simulink library "DiSC_ToolboxOpal_V12"  (R2012b)
settings: Solver=ode45  StartTime=0.0  StopTime=10.0  RelTol=1e-3
undefined symbols (not defined in the file or in its folder): SamplingTime
(part 1 of 5)
settings Model: Creator=mos  LastModifiedBy=smartgrid

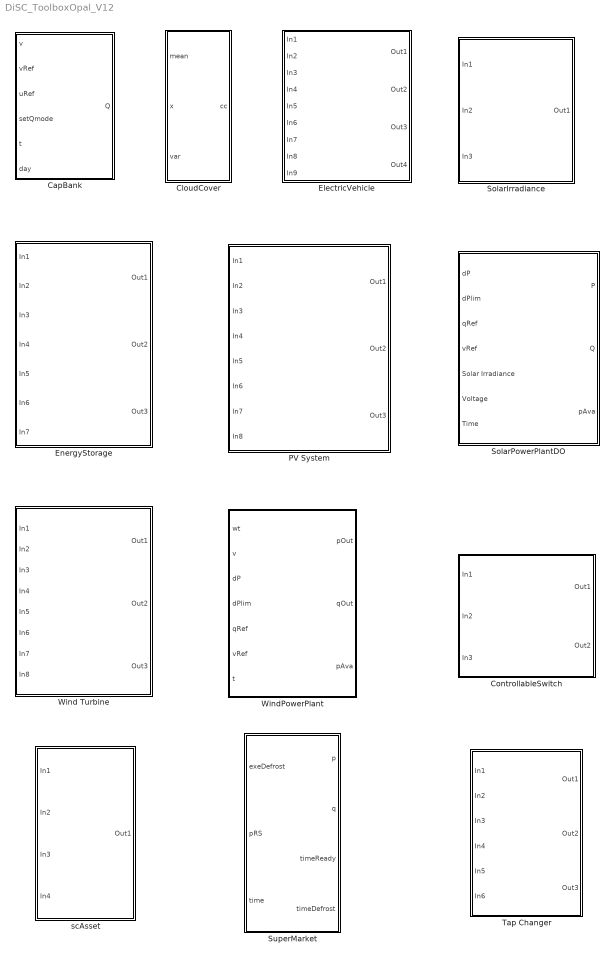
== system DiSC_ToolboxOpal_V12 ==
  CapBank : Subsystem  TreatAsAtomicUnit=on  SystemSampleTime=60
      mask help:
      | % A simulink version of cbAsset module using embedded matlab function
      |     % block on Simulink
      |     %   The cbAsset can be controlled to inject reactive power into the
      |     %   grid in steps. It is characterized by having a number of steps and
      |     %   a reactive output per step (i.e., it can inject from 0 - Qmax in
      |     %   N steps).
      |     %
      |     %
      |     % Revision:
      |     % 15-10-2014, R. Pedersen, Aalborg University. Notes:
      |     % 29-11-2014, R. Olsen/M. Kemal, Aalborg University (Simulink)
      |     % 20-06-2015, F. Iov/M. Kemal, Aalborg University (Simulink toolbox for OPAL)
      |
      |         % Input:
      |             %   - v [V], is the voltage at the connection point.
      |             %   - qRef [VAR], is the reference to active power.
      |             %   - vRef [V], is the voltage reference for the droop control.
      |             %   - uRef [V], is the tap reference
      |             %   - SetQmode will set the reactive power control  mode
      |             %
      |             % Output:
      |             %   - q [VAR], is the reactive power output
      mask Help:
      | % A simulink version of cbAsset module using embedded matlab function
      |     % block on Simulink
      |     %   The cbAsset can be controlled to inject reactive power into the
      |     %   grid in steps. It is characterized by having a number of steps and
      |     %   a reactive output per step (i.e., it can inject from 0 - Qmax in
      |     %   N steps).
      |     %
      |     %
      |     % Revision:
      |     % 15-10-2014, R. Pedersen, Aalborg University. Notes:
      |     % 29-11-2014, R. Olsen/M. Kemal, Aalborg University (Simulink)
      | 
      |         % Input:
      |             %   - v [V], is the voltage at the connection point.
      |             %   - qRef [VAR], is the reference to active power.
      |             %   - vRef [V], is the voltage reference for the droop control.
      |             %
      |             % Output:
      |             %   - q [VAR], is the reactive power output
      mask Display:
      | %%image(imread('cbAsset1.jpg'))
      | port_label('output',1,'q')
      | port_label('input',1,'qRef')
      | port_label('input',2,'vRef')
      | port_label('input',3,'uRef')
      | port_label('input',4,'SetQmode')
      | port_label('input',5,'t')
      | port_label('input',6,'day')
  CloudCover : Subsystem  TreatAsAtomicUnit=on  SystemSampleTime=60
      mask help:
      | %MATLAB embedded block  for OPAL-RT
      |     %
      |     %   The cloud cover model can be used to investigate the behavior
      |     %   of e.g., photovoltaic systems. This model can be used together with
      |     %   the solar irradiance model.
      |     %
      |     %   The model is based on the work by
      |     %   Heinriich Morf (1998-2013)
      |     %
      |     % Revision:
      |     % R. Pedersen, Aalborg University.
      |     % 29-11-2014, R. Olsen/M. Kemal, Aalborg University (Simulink)
      |     % 20-06-2015, F. Iov/M. Kemal, Aalborg University (Simulink toolbox for OPAL)
      mask Help:
      | %MATLAB embedded block  for OPAL-RT
      |     %
      |     %   The cloud cover model can be used to investigate the behavior
      |     %   of e.g., photovoltaic systems. This model can be used together with
      |     %   the solar irradiance model.
      |     %
      |     %   The model is based on the work by
      |     %   Heinriich Morf (1998-2013)
      |     %
      |     % Revision:
      |     % R. Pedersen, Aalborg University.
      |     % 29-11-2014, R. Olsen/M. Kemal, Aalborg University (Simulink)
      |     % 20-06-2015, F. Iov/M. Kemal, Aalborg University (Simulink toolbox for OPAL)
      mask Display:
      | %image(imread('cloudCover.jpg'))
      | port_label('output',1,'cc')
      | port_label('input',1,'mean')
      | port_label('input',2,'var')
      | port_label('input',3,'x')
  ControllableSwitch : Subsystem  TreatAsAtomicUnit=on  SystemSampleTime=60
      mask help:
      | %#codegen
      |     % A Simulink implementation of swAsset using embedded MATLAB function
      |     %%swAsset implements a controllable switch.
      |     %   The swAsset can change the switch position between open and closed.
      |     %   The switch is used to change the electrical grid topology.
      |     %   To ensure realistic simulation scenarios a minimum time between
      |     %   switch state change has been incorporated, along with a maximum
      |     %   number of state changes per day.
      |     %
      |     %   The model is intended for studying voltage control problems and
      |     %   power loss minimization. The switch works by inserting an
      |     %   admittance into the admittance matrix whenever the switch state is
      |     %   closed.
      |     %
      |     % R. Pedersen 05-9-2014, Aalborg University
      |     % 20-06-2015, F. Iov/M. Kemal, Aalborg University (Simulink toolbox for OPAL)
      |     % This template includes the minimum set of functions required
      |     % to define a System object with discrete state.
      |
      |
      |             % Input:
      |             %   - uRef [-], is the reference to switch state (0=open, 1=closed).
      |             %   - k [-], is the sample.
      |             %   - day [-], is the day of the simulation (1-365).
      |             %
      |             % Output:
      |             %   - state [-], is the state of the switch, either open or closed.
      |             %   - y [-], is the admittance to be put into the grid admittance matrix.
      |
      |             % If day changes reset the number of switches a day
      mask Help:
      | %#codegen
      |     % A Simulink implementation of swAsset using embedded MATLAB function
      |     %%swAsset implements a controllable switch.
      |     %   The swAsset can change the switch position between open and closed.
      |     %   The switch is used to change the electrical grid topology.
      |     %   To ensure realistic simulation scenarios a minimum time between
      |     %   switch state change has been incorporated, along with a maximum
      |     %   number of state changes per day.
      |     %
      |     %   The model is intended for studying voltage control problems and
      |     %   power loss minimization. The switch works by inserting an
      |     %   admittance into the admittance matrix whenever the switch state is
      |     %   closed.
      |     %
      |     % R. Pedersen 05-9-2014, Aalborg University
      |     % 20-06-2015, F. Iov/M. Kemal, Aalborg University (Simulink toolbox for OPAL)
      |     % This template includes the minimum set of functions required
      |     % to define a System object with discrete state.
      | 
      | 
      |             % Input:
      |             %   - uRef [-], is the reference to switch state (0=open, 1=closed).
      |             %   - k [-], is the sample.
      |             %   - day [-], is the day of the simulation (1-365).
      |             %
      |             % Output:
      |             %   - state [-], is the state of the switch, either open or closed.
      |             %   - y [-], is the admittance to be put into the grid admittance matrix.
      | 
      |             % If day changes reset the number of switches a day
      mask Display:
      | %image(imread('images\switch.jpg'))
      | port_label('output',1,'state')
      | port_label('output',2,'y')
      | port_label('input',1,'uRef')
      | port_label('input',2,'day')
      | port_label('input',3,'t')
  ElectricVehicle : Subsystem  TreatAsAtomicUnit=on  SystemSampleTime=60
      mask help:
      | % evAsset implements a simple electrical vehicel mobility- and battery model in Simulink.
      |     %   The active power consumption of the battery charging cycle can be
      |     %   controlled when ever the electrical vehical is available at
      |     %   a household charging spot.
      |     %   To simulate when the electrical vehical is available data from the
      |     %   National Travel Survey from Great Britain is used.
      |     %
      |     %   To model the battery a simple first order model of an energy
      |     %   storages is used. The batterys state of charges, when arriving at a
      |     %   charging station/spot, is dependent on the trip the car has conducted.
      |     %
      |     %
      |     % Revision:
      |     % 16-07-2014, C.E. Sloth and R. Pedersen, Aalborg University. Notes:
      |     % 29-11-2014, R. Olsen/M. Kemal, Aalborg University (Simulink)
      |     % 20-06-2015, F. Iov/M. Kemal, Aalborg University (Simulink toolbox for OPAL)
      |             % Input:
      |             %   - k [-], is the sample number.
      |             %   - day [day number], is the day of the year 1-365.
      |             %   - v [-], is the voltage at the connection point.
      |             %   - pRef [W], is the reference to active power.
      |             %   - qRef [VAR], is the reference to reactive power.
      |             %   - vRef [V], is the voltage reference.
      |             %
      |             % Output:
      |             %   - p [W], is the active power output.
      |             %   - q [VAR], is the reactive power output.
      |             %   - e [J], is the EV batery energy level.
      |             %   - away [-]. Indicates if the EV is available for charging.
      |
      |             % If day changes calculate when EV is away from home and how
      |             % much the state of charge has changed.
      mask Help:
      | % evAsset implements a simple electrical vehical mobility- and battery model in Simulink.
      |     %   The active power consumption of the battery charging cycle can be
      |     %   controlled when ever the electrical vehical is available at
      |     %   a household charging spot.
      |     %   To simulate when the electrical vehical is available data from the
      |     %   National Travel Survey from Great Britain is used.
      |     %
      |     %   To model the battery a simple first order model of an energy
      |     %   storages is used. The batterys state of charges, when arriving at a
      |     %   charging station/spot, is dependent on the trip the car has conducted.
      |     %
      |     %
      |     % Revision:
      |     % 16-07-2014, C.E. Sloth and R. Pedersen, Aalborg University. Notes:
      |     % 29-11-2014, R. Olsen/M. Kemal, Aalborg University (Simulink)
      |     % 20-06-2015, F. Iov/M. Kemal, Aalborg University (Simulink toolbox for OPAL)
      |             % Input:
      |             %   - k [-], is the sample number.
      |             %   - day [day number], is the day of the year 1-365.
      |             %   - v [-], is the voltage at the connection point.
      |             %   - pRef [W], is the reference to active power.
      |             %   - qRef [VAR], is the reference to reactive power.
      |             %   - vRef [V], is the voltage reference.
      |             %
      |             % Output:
      |             %   - p [W], is the active power output.
      |             %   - q [VAR], is the reactive power output.
      |             %   - e [J], is the EV batery energy level.
      |             %   - away [-]. Indicates if the EV is available for charging.
      | 
      |             % If day changes calculate when EV is away from home and how
      |             % much the state of charge has changed.
      mask Display:
      | %image(imread( 'electricVehicle.jpg'))
      | port_label( 'output',1, 'p')
      | port_label( 'output',2, 'q')
      | port_label( 'output',3, 'e')
      | port_label( 'output',4, 'away')
      | 
      | port_label( 'input',1, 'day')
      | port_label( 'input',2, 'vMeas')
      | port_label( 'input',3, 'pRef')
      | port_label( 'input',4, 'pMode')
      | port_label( 'input',5, 'qRef')
      | port_label( 'input',6, 'qMode')
      | port_label( 'input',7, 'vRef')
      | port_label( 'input',8, 'time')
      | port_label( 'input',9, 'seed')
  EnergyStorage : Subsystem  TreatAsAtomicUnit=on  SystemSampleTime=60
      mask help:
      | % A Simulink model of esAsset for Simulink using embedded matlab
      |     % function
      |     % esAsset implements a simple controllable energy storage.
      |     %   The esAsset can be set to consume active power or inject active
      |     %   power. The energy storage consumes reactive power with a constant
      |     %   power factor. The energy storage can also be set to do voltage
      |     %   droop control.
      |     %
      |     %
      |     % Revision:
      |     % 23-06-2014, R. Pedersen, Aalborg University. Notes:
      |     % 29-11-2014, R. Olsen/M. Kemal, Aalborg University (Simulink)
      |     % 20-06-2015, F. Iov/M. Kemal, Aalborg University (Simulink toolbox for OPAL)
      |
      |             % Input:
      |             %   - v, is the voltage at the connection point.
      |             %   - pRef, is the reference to active power.
      |             %   - vRef, is the voltage reference for the droop control
      |             %
      |             % Output:
      |             %   - p [W], is the active power consumption
      |             %   - q [VAR], is the reactive power output
      |             %   - e [J], is the energy storage energy level
      mask Help:
      | % A Simulink model of esAsset for Simulink using embedded matlab
      |     % function
      |     % esAsset implements a simple controllable energy storage.
      |     %   The esAsset can be set to consume active power or inject active
      |     %   power. The energy storage consumes reactive power with a constant
      |     %   power factor. The energy storage can also be set to do voltage
      |     %   droop control.
      |     %
      |     %
      |     % Revision:
      |     % 23-06-2014, R. Pedersen, Aalborg University. Notes:
      |     % 29-11-2014, R. Olsen/M. Kemal, Aalborg University (Simulink)
      |     % 20-06-2015, F. Iov/M. Kemal, Aalborg University (Simulink toolbox for OPAL)
      | 
      |             % Input:
      |             %   - v, is the voltage at the connection point.
      |             %   - pRef, is the reference to active power.
      |             %   - vRef, is the voltage reference for the droop control
      |             %
      |             % Output:
      |             %   - p [W], is the active power consumption
      |             %   - q [VAR], is the reactive power output
      |             %   - e [J], is the energy storage energy level
      mask Display:
      | %image(imread( 'energyStorage.jpg'))
      | port_label( 'output',1, 'p')
      | port_label( 'output',2, 'q')
      | port_label( 'output',3, 'e')
      | port_label( 'input',1, 'vMeas')
      | port_label( 'input',2, 'pRef')
      | port_label( 'input',3, 'pMode')
      | port_label( 'input',4, 'qRef')
      | port_label( 'input',5, 'qMode')
      | port_label( 'input',6, 'vRef')
      | port_label( 'input',7, 'time')
  PV System : Subsystem  TreatAsAtomicUnit=on  SystemSampleTime=60
      mask help:
      | %pvAssetDO implements a simple P,Q controllable solar PV system using MATLAB embedded function.
      |     %   The pvAsset can be set to follow an active power reference, output
      |     %   maximum power available or derate power. It can also, at the same
      |     %   time be set to follow a reactive power reference, output the
      |     %   minimum reactive power according to the power factor or try to keep
      |     %   a voltage reference in the coupling point by controlling reactive
      |     %   power output.
      |     %
      |     %
      |     % Revision:
      |     % 19-06-2014, R. Pedersen, Aalborg University. Notes:
      |     % R. Pedersen 11-6-2014, Aalborg University
      |     % 29-11-2014, R. Olsen/M. Kemal, Aalborg University (Simulink)
      |     % 20-06-2015, F. Iov/M. Kemal, Aalborg University (Simulink toolbox for OPAL)
      |
      |                 % Input:
      |             %   - s [w/m^2], is the solar irradiance.
      |             %   - v [V], is the voltage at the connection point.
      |             %   - dP [PU], is the reference to active power change (curtailment).
      |             %   - dPlim [PU], is the reference to derated power (derate)
      |             %   - qRef [VAR], is the reactive power reference.
      |             %   - vRef [V], is the voltage reference.
      |             %
      |             % Output:
      |             %   - p [W], is the active power output
      |             %   - q [VAR], is the reactive power output
      |             %   - pAva [W], is the available power
      mask Help:
      | %pvAssetDO implements a simple P,Q controllable solar PV system using MATLAB embedded function.
      |     %   The pvAsset can be set to follow an active power reference, output
      |     %   maximum power available or derate power. It can also, at the same
      |     %   time be set to follow a reactive power reference, output the
      |     %   minimum reactive power according to the power factor or try to keep
      |     %   a voltage reference in the coupling point by controlling reactive
      |     %   power output.
      |     %
      |     %
      |     % Revision:
      |     % 19-06-2014, R. Pedersen, Aalborg University. Notes:
      |     % R. Pedersen 11-6-2014, Aalborg University
      |     % 29-11-2014, R. Olsen/M. Kemal, Aalborg University (Simulink)
      |     % 20-06-2015, F. Iov/M. Kemal, Aalborg University (Simulink toolbox for OPAL)
      | 
      |                 % Input:
      |             %   - s [w/m^2], is the solar irradiance.
      |             %   - v [V], is the voltage at the connection point.
      |             %   - dP [W], is the reference to active power change.
      |             %   - dPlim [W], is the reference to derated power.
      |             %   - qRef [VAR], is the reactive power reference.
      |             %   - vRef [V], is the voltage reference.
      |             %
      |             % Output:
      |             %   - p [W], is the active power output
      |             %   - q [VAR], is the reactive power output
      |             %   - pAva [W], is the available power
      mask Display:
      | %image(imread( 'PhotoVoltaic.png'))
      | port_label( 'output',1, 'p')
      | port_label( 'output',2, 'q')
      | port_label( 'output',3, 'pAva')
      | port_label( 'input',1, 'solarIrr')
      | port_label( 'input',2, 'vMeas')
      | port_label( 'input',3, 'time')
      | port_label( 'input',4, 'dp')
      | port_label( 'input',5, 'dplim')
      | port_label( 'input',6, 'qRef')
      | port_label( 'input',7, 'qMode')
      | port_label( 'input',8, 'vRef')
  SolarIrradiance : Subsystem  TreatAsAtomicUnit=on  SystemSampleTime=60
      mask help:
      | %solarIrradianceS implements a solar irradiance model using
      |    %MATLAB embedded block of simulink for OPAL-RT
      |     %   The solar irradiance model can be used to investigate the behavior
      |     %   of e.g., photovoltaic systems. The model is based on the work by
      |     %   Heinriich Morf (1998-2013) and the book: "An Introduction to Solar
      |     %   Radiation", 1983.
      |     %
      |     %
      |     % Revision
      |     % R. Pedersen 11-6-2014, Aalborg University
      |     % 29-11-2014, R. Olsen/M. Kemal, Aalborg University (Simulink)
      |     % 20-06-2015, F. Iov/M. Kemal, Aalborg University (Simulink toolbox for OPAL)
      |
      |             % Input:
      |             %   k [-], is the sample number. Used for zenit angle
      |             %   day [-], is the Julian day of the year (1-365)
      |             %   cc [-], is cloud cover (0-1);
      |             %
      |             % Output:
      |             %   Go [w/m^2], is the irradiance on a horizontal surface.
      mask Help:
      | %solarIrradianceS implements a solar irradiance model using
      |    %MATLAB embedded block of simulink for OPAL-RT
      |     %   The solar irradiance model can be used to investigate the behavior
      |     %   of e.g., photovoltaic systems. The model is based on the work by
      |     %   Heinriich Morf (1998-2013) and the book: "An Introduction to Solar
      |     %   Radiation", 1983.
      |     %
      |     %
      |     % Revision
      |     % R. Pedersen 11-6-2014, Aalborg University
      |     % 29-11-2014, R. Olsen/M. Kemal, Aalborg University (Simulink)
      |     % 20-06-2015, F. Iov/M. Kemal, Aalborg University (Simulink toolbox for OPAL)
      | 
      |             % Input:
      |             %   k [-], is the sample number. Used for zenit angle
      |             %   day [-], is the Julian day of the year (1-365)
      |             %   cc [-], is cloud cover (0-1);
      |             %
      |             % Output:
      |             %   Go [w/m^2], is the irradiance on a horizontal surface.
      mask Display:
      | %image(imread('solarIrradiance.png'))
      | port_label('output',1,'Go')
      | port_label('input',1,'day')
      | port_label('input',2,'cc')
      | port_label('input',3,'time')
  SolarPowerPlantDO : Subsystem  TreatAsAtomicUnit=on
      settings: RTWFcnNameOpts=Use subsystem name  RTWFileNameOpts=Use function name
      mask Display:
      | %image(imread( 'PhotoVoltaicPlant.jpg'))
      | port_label( 'output',1, 'p')
      | port_label( 'output',2, 'q')
      | port_label( 'output',3, 'pAva')
      | 
      | 
      | port_label( 'input',1, 'dp')
      | port_label( 'input',2, 'dplim')
      | port_label( 'input',3, 'qRef')
      | port_label( 'input',4, 'vRef')
      | port_label( 'input',5, 'Solar Irradiance')
      | port_label( 'input',6, 'voltage')
      | port_label( 'input',7, 'time')
  SuperMarket : Subsystem  TreatAsAtomicUnit=on  SystemSampleTime=60
      mask help:
      | % Simulink version of supermarket model using embedded MATLAB function
      | %%Supermarket with flexible defrost cycles for demand response purpose
      | %   This class implements a model of a supermarket with flexible
      | %   defrost cycles. The defrost cycles of low temperature display cases
      | %   are allowed to be shifted in time under certain bounds. The reason
      | %   for only using low temperature dispaly cases is that these use
      | %   electrical heating elements for actively melting the ice during
      | %   defrost cycles. These heating elements consume a substantial amount
      | %   of power.
      | %
      | %   For a formal description of supermarket defrost flexibility, see the
      | %   note on the homepage:
      | %   http://kom.aau.dk/project/SmartGridControl/DiSC/documentation.html
      | %
      | % Revision:
      | % 16-07-2014, R. Pedersen, Aalborg University. Notes:
      | % 29-11-2014, R. Olsen/M. Kemal, Aalborg University (Simulink)
      | % 20-06-2015, F. Iov/M. Kemal, Aalborg University (Simulink toolbox for OPAL)
      |
      |             % Implement algorithm. Calculate y as a function of
      |             % input u and discrete states.
      |              % Input:
      |             %   - exeDefrost [-], is the external control signal to execute defrost cycles.
      |             %   - pRS [W], is the power consumption of the refrigeration system, this should be provided as data.
      |             %
      |             % Output:
      |             %   - p [W], is the active power consumption of the supermarket.
      |             %   - q [VAR], is the reactive power consumption of the supermarket.
      |             %   - timeReady [s], is the time until defrost cycles are ready to be executed.
      |             %   - timeDefrost [s], is the time until the defrost cycles will be executed by the supermarket.
      |
      |             % Power and time flexibility from defrost cycle
      mask Help:
      | % Simulink version of supermarket model using embedded MATLAB function
      | %%Supermarket with flexible defrost cycles for demand response purpose
      | %   This class implements a model of a supermarket with flexible
      | %   defrost cycles. The defrost cycles of low temperature display cases
      | %   are allowed to be shifted in time under certain bounds. The reason
      | %   for only using low temperature dispaly cases is that these use
      | %   electrical heating elements for actively melting the ice during
      | %   defrost cycles. These heating elements consume a substantial amount
      | %   of power.
      | %
      | %   For a formal description of supermarket defrost flexibility, see the
      | %   note on the homepage:
      | %   http://kom.aau.dk/project/SmartGridControl/DiSC/documentation.html
      | %
      | % Revision:
      | % 16-07-2014, R. Pedersen, Aalborg University. Notes:
      | % 29-11-2014, R. Olsen/M. Kemal, Aalborg University (Simulink)
      | % 20-06-2015, F. Iov/M. Kemal, Aalborg University (Simulink toolbox for OPAL)
      | 
      |             % Implement algorithm. Calculate y as a function of
      |             % input u and discrete states.
      |              % Input:
      |             %   - exeDefrost [-], is the external control signal to execute defrost cycles.
      |             %   - pRS [W], is the power consumption of the refrigeration system, this should be provided as data.
      |             %
      |             % Output:
      |             %   - p [W], is the active power consumption of the supermarket.
      |             %   - q [VAR], is the reactive power consumption of the supermarket.
      |             %   - timeReady [s], is the time until defrost cycles are ready to be executed.
      |             %   - timeDefrost [s], is the time until the defrost cycles will be executed by the supermarket.
      | 
      |             % Power and time flexibility from defrost cycle
      mask Display:
      | %image(imread( 'supermarket.jpg'))
      | % port_label( 'output',1, 'Out1')
      | % port_label( 'output',2, 'Out2')
      | % port_label( 'output',3, 'Out3')
      | % port_label( 'output',4, 'Out4')
      | %
      | %
      | % port_label( 'input',1, 'In1')
      | % port_label( 'input',2, 'In2')
      | % port_label( 'input',3, 'In3')
  Tap Changer : Subsystem  TreatAsAtomicUnit=on  SystemSampleTime=60
      mask help:
      | %tcAssetDO implements a controllable tap changing transformer using
      |    %MATLAB embedded block of simulink
      |    %
      |    %
      |     %   The tcAsset can change the tap position of a transformer and
      |     %   thereby effectively change the transformers ratio.
      |     %   The tap changer can be used to simulate e.g., an on-load tap changing
      |     %   transformer. The tap changer works by altering the grid admittance
      |     %   matrix, when ever the tap position is changed. To ensure realistic
      |     %   simulation scenarios a minimum time between tap changes has been
      |     %   incorporated, along with a specified maximum number of tap changes
      |     %   per day.
      |     %
      |     %   The model is intended for studing voltage control problems and can
      |     %   be set to run in two different modes; follow tap reference and
      |     %   apply voltage control. The model is based on the one found in "Power Systems
      |     %   Stability and Control, P. Kundur".
      |     %
      |     % Revision:
      |     % 03-09-2014, R. Pedersen, Aalborg University. Notes:
      |     % 29-11-2014, R. Olsen/M. Kemal, Aalborg University (Simulink)
      |     % 20-06-2015, F. Iov/M. Kemal, Aalborg University (Simulink toolbox for OPAL)
      |             % Input:
      |             %   - v, is the voltage at the connection point.
      |             %   - vRef, is the voltage reference for the voltage
      |             %     control.
      |             %   - uRef, is the reference to tap position.
      |             %   - k, is the sample.
      |             %   - day, is the day of the simulation (1-365).
      |             %
      |             % Output:
      |             %   - y1, y2, y3, is the transformer admittances between busses,
      |             %     from ground to primary side bus and from ground to
      |             %     secondary side bus, respectively.
      mask Help:
      | %tcAssetDO implements a controllable tap changing transformer using
      |    %MATLAB embedded block of simulink
      |    %
      |    %
      |     %   The tcAsset can change the tap position of a transformer and
      |     %   thereby effectively change the transformers ratio.
      |     %   The tap changer can be used to simulate e.g., an on-load tap changing
      |     %   transformer. The tap changer works by altering the grid admittance
      |     %   matrix, when ever the tap position is changed. To ensure realistic
      |     %   simulation scenarios a minimum time between tap changes has been
      |     %   incorporated, along with a specified maximum number of tap changes
      |     %   per day.
      |     %
      |     %   The model is intended for studing voltage control problems and can
      |     %   be set to run in two different modes; follow tap reference and
      |     %   apply voltage control. The model is based on the one found in "Power Systems
      |     %   Stability and Control, P. Kundur".
      |     %
      |     % Revision:
      |     % 03-09-2014, R. Pedersen, Aalborg University. Notes:
      |     % 29-11-2014, R. Olsen/M. Kemal, Aalborg University (Simulink)
      |     % 20-06-2015, F. Iov/M. Kemal, Aalborg University (Simulink toolbox for OPAL)
      |             % Input:
      |             %   - v, is the voltage at the connection point.
      |             %   - vRef, is the voltage reference for the voltage
      |             %     control.
      |             %   - uRef, is the reference to tap position.
      |             %   - k, is the sample.
      |             %   - day, is the day of the simulation (1-365).
      |             %
      |             % Output:
      |             %   - y1, y2, y3, is the transformer admittances between busses,
      |             %     from ground to primary side bus and from ground to
      |             %     secondary side bus, respectively.
      mask Display:
      | %image(imread( 'tapChanger.jpg'))
      | port_label( 'output',1, 'y1')
      | port_label( 'output',2, 'y2')
      | port_label( 'output',3, 'y3')
      | 
      | 
      | port_label( 'input',1, 'vMeas')
      | port_label( 'input',2, 'vRef')
      | port_label( 'input',3, 'uRef')
      | port_label( 'input',4, 'mode')
      | port_label( 'input',5, 'day')
      | port_label( 'input',6, 'time')
  Wind Turbine : Subsystem
      mask help:
      | %wtAssetS implements a simple P,Q controllable wind turbine system for Simulink.
      |     % This model works for Simulink and requires generatedWindFiles to
      |     % have been executed before running the simulink model
      |     %
      |     %   The wtAsset can be set to follow an active power reference, output
      |     %   maximum power available or curtail power. It can also, at the same
      |     %   time be set to follow a reactive power reference, output the
      |     %   minimum reactive power according to the power factor or try to keep
      |     %   a voltage reference in the coupling point by controlling reactive
      |     %   power output.
      |     %
      |     %   The model is partly based on the book
      |     %   "Optimal Control of Wind Energy Systems 2008".
      |     %
      |     %
      |     % Revision:
      |     % 23-05-2014, C. E. Sloth and R. Pedersen, Aalborg University. Notes:
      |     % 29-11-2014, R. Olsen/M. Kemal, Aalborg University (Simulink)
      |     % 20-06-2015, F. Iov/M. Kemal, Aalborg University (Simulink toolbox for OPAL)
      |             % Input:
      |             %   - w [m/s], is the wind speed.
      |             %   - v [PU], is the voltage at the connection point.
      |             %   - dP [PU], is the reference to active power change (curtailment).
      |             %   - dPlim [PU], is the reference to derated power (derate).
      |             %   - qRef [PU], is the reactive power reference.
      |             %   - vRef [PU], is the voltage reference.
      |             %
      |             % Output:
      |             %   - p [W], is active power outpur.
      |             %   - q [VAR], is reactive power output.
      |             %   - pAva [W], is the available active power
      mask Help:
      | %wtAssetS implements a simple P,Q controllable wind turbine system for Simulink.
      |     % This model works for Simulink and requires generatedWindFiles to
      |     % have been executed before running the simulink model
      |     %
      |     %   The wtAsset can be set to follow an active power reference, output
      |     %   maximum power available or curtail power. It can also, at the same
      |     %   time be set to follow a reactive power reference, output the
      |     %   minimum reactive power according to the power factor or try to keep
      |     %   a voltage reference in the coupling point by controlling reactive
      |     %   power output.
      |     %
      |     %   The model is partly based on the book
      |     %   "Optimal Control of Wind Energy Systems 2008".
      |     %
      |     %
      |     % Revision:
      |     % 23-05-2014, C. E. Sloth and R. Pedersen, Aalborg University. Notes:
      |     % 29-11-2014, R. Olsen/M. Kemal, Aalborg University (Simulink)
      |     % 20-06-2015, F. Iov/M. Kemal, Aalborg University (Simulink toolbox for OPAL)
      |             % Input:
      |             %   - w [m/s], is the wind speed.
      |             %   - v [PU], is the voltage at the connection point.
      |             %   - dP [PU], is the reference to active power change (curtailment).
      |             %   - dPlim [PU], is the reference to derated power (derate).
      |             %   - qRef [PU], is the reactive power reference.
      |             %   - vRef [PU], is the voltage reference.
      |             %
      |             % Output:
      |             %   - p [W], is active power outpur.
      |             %   - q [VAR], is reactive power output.
      |             %   - pAva [W], is the available active power
      mask Display:
      | %image(imread( 'windTurbine.jpg'))
      | port_label( 'output',1, 'p')
      | port_label( 'output',2, 'q')
      | port_label( 'output',3, 'pAva')
      | 
      | 
      | port_label( 'input',1, 'wind')
      | port_label( 'input',2, 'vMeas')
      | port_label( 'input',3, 'dp')
      | port_label( 'input',4, 'dplim')
      | port_label( 'input',5, 'qRef')
      | port_label( 'input',6, 'qMode')
      | port_label( 'input',7, 'vRef')
      | port_label( 'input',8, 'time')
  WindPowerPlant : Subsystem  TreatAsAtomicUnit=on  SystemSampleTime=60
      settings: RTWFcnNameOpts=Use subsystem name  RTWFileNameOpts=Use function name
      mask Display: %image(imread( 'windPowerPlant.jpg'))
  scAsset : Subsystem  TreatAsAtomicUnit=on  SystemSampleTime=60
      mask help:
      | % A Simulink model of SC Asset using MATLAB embedded function block of simulink
      |     % %scAsset implements a simple controllable static compensator asset.
      |     %   The scAsset can be set to inject or consume reactive power based
      |     %   on a reference  or do voltage droop control.
      |     %
      |     %   This model is based on a simple algebraic principle, as it is
      |     %   intended for sampling times higher than 1 second.
      |     %
      |     % Revision:
      |     % 23-06-2014, R. Pedersen, Aalborg University. Notes:
      |     % 29-11-2014, R. Olsen/M. Kemal, Aalborg University (Simulink)
      |     % 20-06-2015, F. Iov/M. Kemal, Aalborg University (Simulink toolbox for OPAL)
      |
      |                 % Input:
      |             %   - v [V], is the voltage magnitude on the bus.
      |             %   - qRef [VAR], is the reference to reactive power.
      |             %   - vRef [V], is the voltage reference.
      |             %
      |             % Output:
      |             %   - q [VAR], reactive power output.
      mask Help:
      | % A Simulink model of SC Asset using MATLAB embedded function block of simulink
      |     % %scAsset implements a simple controllable static compensator asset.
      |     %   The scAsset can be set to inject or consume reactive power based
      |     %   on a reference  or do voltage droop control.
      |     %
      |     %   This model is based on a simple algebraic principle, as it is
      |     %   intended for sampling times higher than 1 second.
      |     %
      |     % Revision:
      |     % 23-06-2014, R. Pedersen, Aalborg University. Notes:
      |     % 29-11-2014, R. Olsen/M. Kemal, Aalborg University (Simulink)
      |     % 20-06-2015, F. Iov/M. Kemal, Aalborg University (Simulink toolbox for OPAL)
      | 
      |                 % Input:
      |             %   - v [V], is the voltage magnitude on the bus.
      |             %   - qRef [VAR], is the reference to reactive power.
      |             %   - vRef [V], is the voltage reference.
      |             %
      |             % Output:
      |             %   - q [VAR], reactive power output.
      mask Display:
      | %image(imread('staticCompensator.jpg'))
      | port_label('output',1,'q')
      | port_label('input',1,'v')
      | port_label('input',2,'qRef')
      | port_label('input',3,'vRef')
      | port_label('input',4,'t')

== system DiSC_ToolboxOpal_V12/CapBank ==
  v : Inport
  vRef : Inport  Port=2
  uRef : Inport  Port=3
  setQmode : Inport  Port=4
  t : Inport  Port=5
  day : Inport  Port=6
  MATLAB Function : MATLAB Function  TreatAsAtomicUnit=on  SystemSampleTime=SamplingTime
  Q : Outport
  wires:
  setQmode/1 -> MATLAB Function/4(setQmode)
  v/1 -> MATLAB Function/1(v)
  MATLAB Function/1(q) -> Q/1
  t/1 -> MATLAB Function/5(t)
  day/1 -> MATLAB Function/6(day)
  vRef/1 -> MATLAB Function/2(vRef)
  uRef/1 -> MATLAB Function/3(uRef)

== system DiSC_ToolboxOpal_V12/CloudCover ==
  mean : Inport
  x : Inport  Port=2
  var : Inport  Port=3
  MATLAB Function1 : MATLAB Function  TreatAsAtomicUnit=on
  cc : Outport
  wires:
  var/1 -> MATLAB Function1/2(var)
  mean/1 -> MATLAB Function1/1(mean)
  MATLAB Function1/1(cc) -> cc/1
  x/1 -> MATLAB Function1/3(x)

== system DiSC_ToolboxOpal_V12/ControllableSwitch ==
  In1 : Inport
  In2 : Inport  Port=2
  In3 : Inport  Port=3
  MATLAB Function : MATLAB Function  TreatAsAtomicUnit=on
  Out1 : Outport
  Out2 : Outport  Port=2
  wires:
  In1/1 -> MATLAB Function/1(uRef)
  In2/1 -> MATLAB Function/2(day)
  MATLAB Function/2(y) -> Out2/1
  In3/1 -> MATLAB Function/3(t)
  MATLAB Function/1(state) -> Out1/1

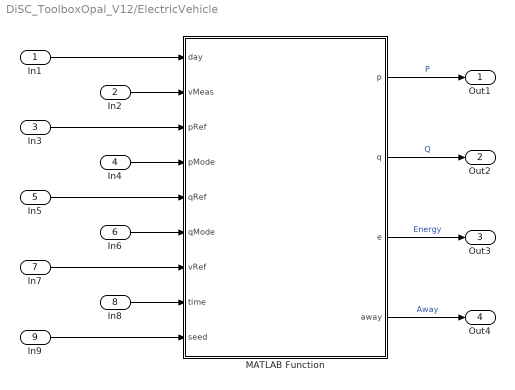
== system DiSC_ToolboxOpal_V12/ElectricVehicle ==
  In1 : Inport
  In2 : Inport  Port=2
  In3 : Inport  Port=3
  In4 : Inport  Port=4
  In5 : Inport  Port=5
  In6 : Inport  Port=6
  In7 : Inport  Port=7
  In8 : Inport  Port=8
  In9 : Inport  Port=9
  MATLAB Function : MATLAB Function  TreatAsAtomicUnit=on
  Out1 : Outport
  Out2 : Outport  Port=2
  Out3 : Outport  Port=3
  Out4 : Outport  Port=4
  wires:
  MATLAB Function/1(p) -> Out1/1  "P"
  MATLAB Function/2(q) -> Out2/1  "Q"
  In1/1 -> MATLAB Function/1(day)
  In3/1 -> MATLAB Function/3(pRef)
  In4/1 -> MATLAB Function/4(pMode)
  In8/1 -> MATLAB Function/8(time)
  In9/1 -> MATLAB Function/9(seed)
  In7/1 -> MATLAB Function/7(vRef)
  In5/1 -> MATLAB Function/5(qRef)
  In6/1 -> MATLAB Function/6(qMode)
  MATLAB Function/3(e) -> Out3/1  "Energy"
  MATLAB Function/4(away) -> Out4/1  "Away"
  In2/1 -> MATLAB Function/2(vMeas)

== system DiSC_ToolboxOpal_V12/EnergyStorage ==
  In1 : Inport
  In2 : Inport  Port=2
  In3 : Inport  Port=3
  In4 : Inport  Port=4
  In5 : Inport  Port=5
  In6 : Inport  Port=6
  In7 : Inport  Port=7
  MATLAB Function : MATLAB Function  TreatAsAtomicUnit=on
  Out1 : Outport
  Out2 : Outport  Port=2
  Out3 : Outport  Port=3
  wires:
  In2/1 -> MATLAB Function/2(pRef)
  In5/1 -> MATLAB Function/5(qMode)
  In6/1 -> MATLAB Function/6(vRef)
  MATLAB Function/2(q) -> Out2/1
  In4/1 -> MATLAB Function/4(qRef)
  In7/1 -> MATLAB Function/7(time)
  In3/1 -> MATLAB Function/3(pMode)
  MATLAB Function/1(p) -> Out1/1
  MATLAB Function/3(e) -> Out3/1
  In1/1 -> MATLAB Function/1(vMeas)

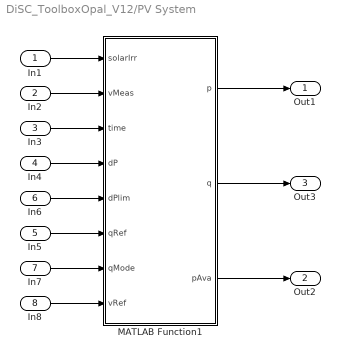
== system DiSC_ToolboxOpal_V12/PV System ==
  In1 : Inport
  In2 : Inport  Port=2
  In3 : Inport  Port=3
  In4 : Inport  Port=4
  In5 : Inport  Port=5
  In6 : Inport  Port=6
  In7 : Inport  Port=7
  In8 : Inport  Port=8
  MATLAB Function1 : MATLAB Function  TreatAsAtomicUnit=on
  Out1 : Outport
  Out2 : Outport  Port=2
  Out3 : Outport  Port=3
  wires:
  In7/1 -> MATLAB Function1/7(qMode)
  In8/1 -> MATLAB Function1/8(vRef)
  MATLAB Function1/2(q) -> Out3/1
  In1/1 -> MATLAB Function1/1(solarIrr)
  In3/1 -> MATLAB Function1/3(time)
  In6/1 -> MATLAB Function1/5(dPlim)
  In4/1 -> MATLAB Function1/4(dP)
  In2/1 -> MATLAB Function1/2(vMeas)
  MATLAB Function1/1(p) -> Out1/1
  In5/1 -> MATLAB Function1/6(qRef)
  MATLAB Function1/3(pAva) -> Out2/1

== system DiSC_ToolboxOpal_V12/SolarIrradiance ==
  In1 : Inport
  In2 : Inport  Port=2
  In3 : Inport  Port=3
  MATLAB Function : MATLAB Function  TreatAsAtomicUnit=on
  Out1 : Outport
  wires:
  In3/1 -> MATLAB Function/3(time)
  MATLAB Function/1(Go) -> Out1/1
  In2/1 -> MATLAB Function/2(cc)
  In1/1 -> MATLAB Function/1(day)
